simulink library "relay_tripOutMng_lib"  (Simulink 8.1)
settings: Solver=ode45  StartTime=0.0  StopTime=10.0  RelTol=1e-3
libraries: simulink x1, simulink_extras x1
settings Model: Creator=RE25624  LastModifiedBy=re25624

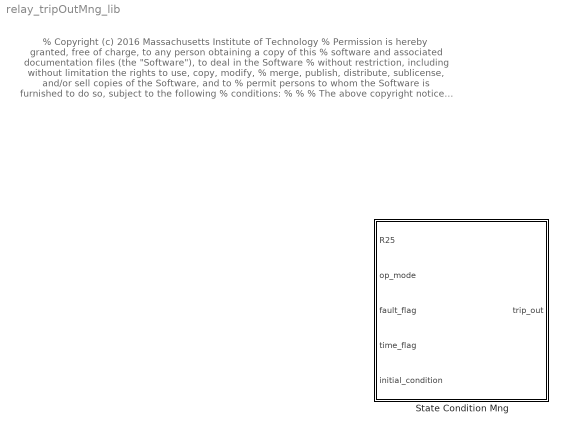
== system relay_tripOutMng_lib ==
  note: % Copyright (c) 2016 Massachusetts Institute of Technology
      | % Permission is hereby granted, free of charge, to any person obtaining a copy of this
      | % software and associated documentation files (the "Software"), to deal in the Software
      | % without restriction, including without limitation the rights to use, copy, modify,
      | % merge, publish, distribute, sublicense, and/or sell copies of the Software, and to
      | % permit persons to whom the Software is furnished to do so, subject to the following
      | % conditions:
      | %
      | %
      | % The above copyright notice and this permission notice shall be included in
      | % all copies or substantial portions of the Software.
      | %
      | % THE SOFTWARE IS PROVIDED "AS IS", WITHOUT WARRANTY OF ANY KIND, EXPRESS OR IMPLIED,
      | % INCLUDING BUT NOT LIMITED TO THE WARRANTIES OF MERCHANTABILITY, FITNESS FOR A
      | % PARTICULAR PURPOSE AND NONINFRINGEMENT. IN NO EVENT SHALL THE AUTHORS OR COPYRIGHT
      | % HOLDERS BE LIABLE FOR ANY CLAIM, DAMAGES OR OTHER LIABILITY, WHETHER IN AN ACTION
      | % OF CONTRACT, TORT OR OTHERWISE, ARISING FROM, OUT OF OR IN CONNECTION WITH THE
      | % SOFTWARE OR THE USE OR OTHER DEALINGS IN THE SOFTWARE.
      | %
      | %
      | %%
  State Condition Mng : Subsystem

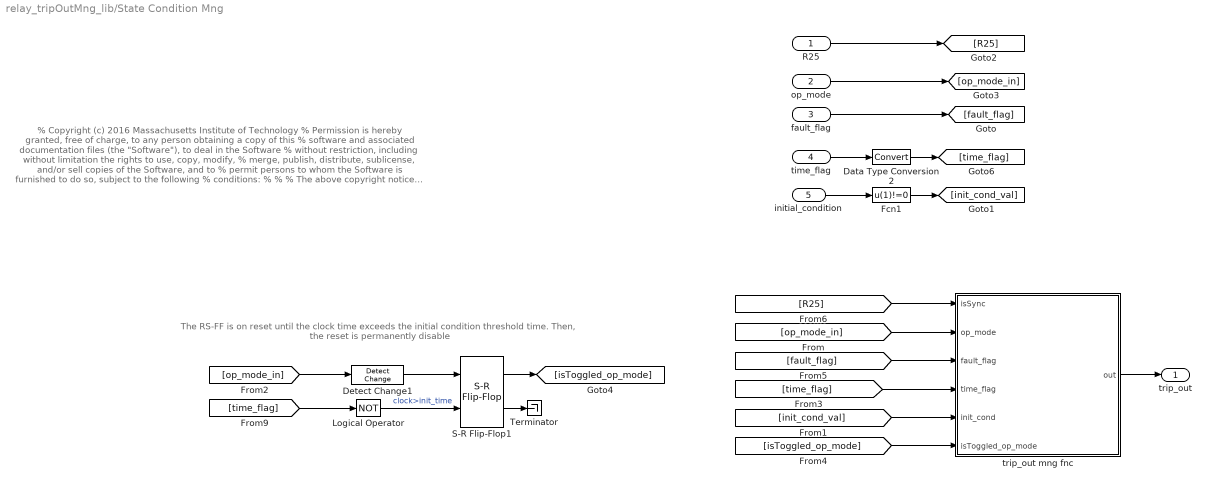
== system relay_tripOutMng_lib/State Condition Mng ==
  note: The RS-FF is on reset until the clock time exceeds the initial condition threshold time.
      | Then, the reset is permanently disable
  note: % Copyright (c) 2016 Massachusetts Institute of Technology
      | % Permission is hereby granted, free of charge, to any person obtaining a copy of this
      | % software and associated documentation files (the "Software"), to deal in the Software
      | % without restriction, including without limitation the rights to use, copy, modify,
      | % merge, publish, distribute, sublicense, and/or sell copies of the Software, and to
      | % permit persons to whom the Software is furnished to do so, subject to the following
      | % conditions:
      | %
      | %
      | % The above copyright notice and this permission notice shall be included in
      | % all copies or substantial portions of the Software.
      | %
      | % THE SOFTWARE IS PROVIDED "AS IS", WITHOUT WARRANTY OF ANY KIND, EXPRESS OR IMPLIED,
      | % INCLUDING BUT NOT LIMITED TO THE WARRANTIES OF MERCHANTABILITY, FITNESS FOR A
      | % PARTICULAR PURPOSE AND NONINFRINGEMENT. IN NO EVENT SHALL THE AUTHORS OR COPYRIGHT
      | % HOLDERS BE LIABLE FOR ANY CLAIM, DAMAGES OR OTHER LIABILITY, WHETHER IN AN ACTION
      | % OF CONTRACT, TORT OR OTHERWISE, ARISING FROM, OUT OF OR IN CONNECTION WITH THE
      | % SOFTWARE OR THE USE OR OTHER DEALINGS IN THE SOFTWARE.
      | %
      | %
      | %%
  R25 : Inport
  op_mode : Inport  Port=2
  fault_flag : Inport  Port=3
  time_flag : Inport  Port=4
  initial_condition : Inport  Port=5
  Data Type Conversion2 : DataTypeConversion
  Detect Change1 : simulink/Logic and Bit Operations/Detect Change  vinit=0  InputProcessing=Inherited  OutDataTypeStr=boolean
  Fcn1 : Fcn  Expr=u(1)!=0
  Logical Operator : Logic  Operator=NOT  AllPortsSameDT=off  OutDataTypeStr=boolean
  S-R Flip-Flop1 : simulink_extras/Flip Flops/S-R Flip-Flop  initial_condition=0
  Terminator : Terminator
  trip_out mng fnc : MATLAB Function  TreatAsAtomicUnit=on
  trip_out : Outport
  wires:
  Data Type Conversion2/1 -> [time_flag]
  Logical Operator/1 -> S-R Flip-Flop1/2  "clock>init_time"
  [time_flag] -> Logical Operator/1
  [time_flag] -> trip_out mng fnc/4(time_flag)
  [isToggled_op_mode] -> trip_out mng fnc/6(isToggled_op_mode)
  S-R Flip-Flop1/1 -> [isToggled_op_mode]
  Detect Change1/1 -> S-R Flip-Flop1/1
  fault_flag/1 -> [fault_flag]
  [fault_flag] -> trip_out mng fnc/3(fault_flag)
  trip_out mng fnc/1(out) -> trip_out/1
  op_mode/1 -> [op_mode_in]
  time_flag/1 -> Data Type Conversion2/1
  [op_mode_in] -> trip_out mng fnc/2(op_mode)
  [R25] -> trip_out mng fnc/1(isSync)
  R25/1 -> [R25]
  [op_mode_in] -> Detect Change1/1
  S-R Flip-Flop1/2 -> Terminator/1
  initial_condition/1 -> Fcn1/1
  [init_cond_val] -> trip_out mng fnc/5(init_cond)
  Fcn1/1 -> [init_cond_val]

== matlab function State Condition Mng/trip_out mng fnc ==
  data: isSync input double; op_mode input double; out output double; fault_flag input double; time_flag input double; init_cond input double; isToggled_op_mode input double
% Copyright (c) 2016 Massachusetts Institute of Technology
% Permission is hereby granted, free of charge, to any person obtaining a copy of this
% software and associated documentation files (the "Software"), to deal in the Software
% without restriction, including without limitation the rights to use, copy, modify,
% merge, publish, distribute, sublicense, and/or sell copies of the Software, and to
% permit persons to whom the Software is furnished to do so, subject to the following
% conditions:
%
%
% The above copyright notice and this permission notice shall be included in
% all copies or substantial portions of the Software.
%
% THE SOFTWARE IS PROVIDED "AS IS", WITHOUT WARRANTY OF ANY KIND, EXPRESS OR IMPLIED,
% INCLUDING BUT NOT LIMITED TO THE WARRANTIES OF MERCHANTABILITY, FITNESS FOR A
% PARTICULAR PURPOSE AND NONINFRINGEMENT. IN NO EVENT SHALL THE AUTHORS OR COPYRIGHT
% HOLDERS BE LIABLE FOR ANY CLAIM, DAMAGES OR OTHER LIABILITY, WHETHER IN AN ACTION
% OF CONTRACT, TORT OR OTHERWISE, ARISING FROM, OUT OF OR IN CONNECTION WITH THE
% SOFTWARE OR THE USE OR OTHER DEALINGS IN THE SOFTWARE.
%
%
%%

function out = opModeChk(isSync, op_mode, fault_flag, time_flag, init_cond, isToggled_op_mode)
%#codegen

% true when simulation time is greater than initial condition time
% time_flag = (clock_time > init_cond_time);
% true when "closed" initial condition and the controller toggles the relay
% operation mode to activate the logic on a "close" cmd. Basically, if the controller
% cmds the relay to close and the relay was already closed.
ctrl_on_flag = (init_cond == 1 && isToggled_op_mode == 1 && (op_mode == 0 || op_mode == 1));
% true when controller cmds the relay to close and logic is active
close_cmd_flag = ((op_mode == 0 || op_mode == 1) && isToggled_op_mode == 1);

if time_flag && fault_flag==0 && isSync==1 && (ctrl_on_flag || close_cmd_flag)
    % true when there is not faults in the relay protection zone, the
    % sync-check is active, and above flags are true
    out = 1; % close cb cmd
elseif time_flag && (fault_flag == 1 || isSync == 0 || op_mode == 2)
    % true when simulation time is greater than initial condition time and
    % there is a fault in the protection zone, or fails to sync, or ctrl cmd
    out = 0; % open cb cmd
else
    out = init_cond;
end
